simulink model "e_ec_u"  (R2014b)
settings: Solver=ode3  StartTime=0.0  StopTime=4  FixedStep=0.0001  RelTol=1e-3
PreLoadFcn:
  | VarName=readfis('e_ec_u.fis');
libraries: fuzblock x1
settings Model: Creator=JRCHAN  LastModifiedBy=JRCHAN
settings OptimizationCC: BooleanDataType=off

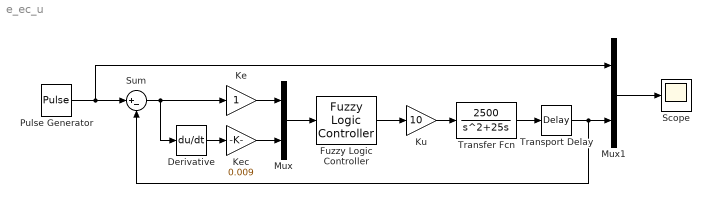
== system e_ec_u ==
  Derivative : Derivative
  Fuzzy Logic Controller : fuzblock/Fuzzy Logic  Controller  fis=[VarName]
  Ke : Gain
  Kec : Gain  Gain=0.009
  Ku : Gain  Gain=10
  Mux : Mux  Inputs=2
  Mux1 : Mux  Inputs=2
  Pulse Generator : DiscretePulseGenerator  PulseType=Time based  Period=1  PulseWidth=50
  Scope : Scope
      settings: TimeRange=5  YMin=-0.4  YMax=2
  Sum : Sum  Inputs=|+-
  Transfer Fcn : TransferFcn  Numerator=[2500]  Denominator=[1 25 0]
  Transport Delay : TransportDelay  DelayTime=0.002
  wires:
  Transfer Fcn/1 -> Transport Delay/1
  Pulse Generator/1 -> Mux1/1, Sum/1
  Sum/1 -> Derivative/1, Ke/1
  Derivative/1 -> Kec/1
  Mux/1 -> Fuzzy Logic Controller/1
  Fuzzy Logic Controller/1 -> Ku/1
  Transport Delay/1 -> Sum/2, Mux1/2
  Mux1/1 -> Scope/1
  Ke/1 -> Mux/1
  Kec/1 -> Mux/2
  Ku/1 -> Transfer Fcn/1
